simulink library "tqd"  (R2021b)
settings: Solver=VariableStepAuto  StartTime=0.0  StopTime=10.0  RelTol=1e-3
undefined symbols (not defined in the file or in its folder): ATQD_APSDecReq_X_kph, ATQD_APSDecReq_Y_mps2, ATQD_APSDecReqCMD_X_kph, ATQD_APSDecReqTs_X_pct, ATQD_APSDecTimeGain_X_Deg, ATQD_APSDecTimeGain_Y_s, ATQD_APSReqLowSpd_X_Deg, ATQD_AutoHoldReleaseBPS_X_Deg, ATQD_AWDLoadTrqnsGain_X_kg, ATQD_AWDLoadTrqnsGain_Y_pct, ATQD_BOSEnBPSPosn_X_kph, ATQD_BOSMap_X_rpm, ATQD_BOSMap_Y_pct, ATQD_CreepBaseTqD_X_kph, ATQD_CreepBaseTqD_Y_Deg, ATQD_CreepBaseTqR_X_kph, ATQD_CreepBaseTqR_Y_Deg, ATQD_CreepBPSDisPosn_X_Deg, ATQD_CreepBPSDisPosnR_X_Deg, ATQD_CreepBPSEnPosn_X_Deg, ATQD_CreepBPSEnPosnR_X_Deg, ATQD_CreepDeltaTq_X_kph, ATQD_CreepIterm_X_kph, ATQD_CreepIterm_Y_kph, ATQD_CreepItermMaxLimit_X_pct, ATQD_CreepPreloadTime_X_kph, ATQD_CreepPreloadTq_X_kph, ATQD_CreepPreloadTq_Y_s, ATQD_CreepProtTq_X_Deg, ATQD_CreepPterm_X_kph, ATQD_ECOTqMapD_X_rpm, ATQD_ECOTqMapD_Y_pct, ATQD_EOPDTqMapDCon_X_rpm, ATQD_EOPDTqMapDCon_Y_Deg, ATQD_EstInitVehWeight_X_c, ATQD_LHMRollGenMapD_X_rpm, ATQD_LHMRollGenMapD_Y_rpm, ATQD_LHMTqMapD_X_rpm, ATQD_LHMTqMapD_Y_pct, ATQD_NL1TqMapD_X_rpm, ATQD_NL1TqMapD_Y_pct, ATQD_NOPDTqMapDCon_X_rpm, ATQD_NOPDTqMapDCon_Y_Deg, ATQD_NRMRrEDUSpRat_X_rpm, ATQD_NRMRrEDUSpRat_Y_Nm, ATQD_OPDHoldDownRelDelay_X_Deg, ATQD_OPDHoldEnSpd_X_Deg, ATQD_OPDHoldRelDetTime_X_Deg, ATQD_OPDHoldReleaseTq_X_Deg, ATQD_OrigPedTqLowLim_X_Deg, ATQD_OrigPedTqLowLim_Y_pct, ATQD_PedalMapClimbUpLim_X_rpm, ATQD_PedalMapClimbUpLim_Y_Deg, ATQD_PreLoadTq_X_s, ATQD_RollGenMapEL1_X_rpm, ATQD_RollGenMapEL1_Y_rpm, ATQD_SL1TqMapD_X_rpm, ATQD_SL1TqMapD_Y_pct, ATQD_SlideRegenTqGain_X_Gps, ATQD_SlideRegenTqGain_Y_pct ... (+444)
libraries: hcu_lib x70, simulink x61, tqr x1
(part 10 of 14)

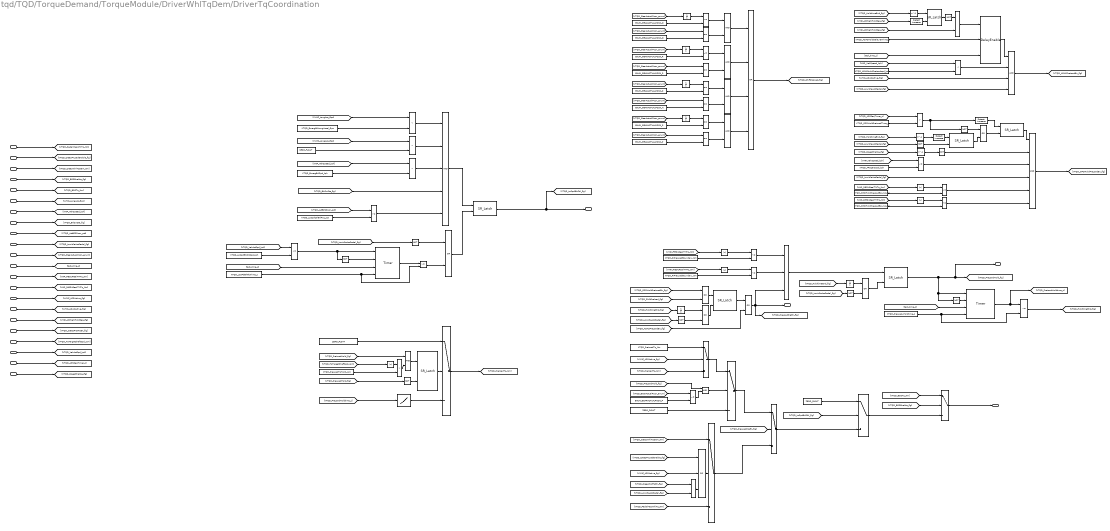
== system tqd/TQD/TorqueDemand/TorqueModule/DriverWhlTqDem/DriverTqCoordination ==
  VTQD_PedalMapWhlTq_Nm : Inport
  VTQD_CreepPrLoadEnable_flg : Inport  Port=2
  VTQD_CreepWhlTqDem_Nm : Inport  Port=3
  VTQD_BOSEnable_flg : Inport  Port=4
  VTQD_BOSTq_Nm : Inport  Port=5
  VVMC_LongAcc_Gps : Inport  Port=6
  VINP_VehSpeed_kph : Inport  Port=7
  VTQD_BrkSwSta_flg : Inport  Port=8
  VTQD_ActBPSPosn_pct : Inport  Port=9
  VTQD_LowIdleAccPedal_flg : Inport  Port=10
  VTQD_GearActualPosn_enum : Inport  Port=11
  task_time_s : Inport  Port=12
  VINP_FrEDURealTMTq_Nm : Inport  Port=13
  VINP_RrEDURealTMTq_Nm : Inport  Port=14
  VVMC_APSActive_flg : Inport  Port=15
  VVMC_ADASActive_flg : Inport  Port=16
  VINP_ACCVehHoldReq_flg : Inport  Port=17
  VTQD_CreepProtTqEn_flg : Inport  Port=18
  VTQD_TqTargetShaftSpd_rpm : Inport  Port=19
  VTQD_VehActSpd_kph : Inport  Port=20
  VTQD_APSReqTimer_s : Inport  Port=21
  VTQD_CreepEnable_flg : Inport  Port=22
  AND : Logic  Inputs=3  AllPortsSameDT=off  OutDataTypeStr=boolean
  AND{1..3,7..10} (7 alike) : Logic  AllPortsSameDT=off  OutDataTypeStr=boolean
  AND4 : Logic  Inputs=6  AllPortsSameDT=off  OutDataTypeStr=boolean
  AND5 : Logic  Inputs=4  AllPortsSameDT=off  OutDataTypeStr=boolean
  AND6 : Logic  Inputs=5  AllPortsSameDT=off  OutDataTypeStr=boolean
  Abs{,1..4} (5 alike) : Abs
  Constant : Constant  Value=KTQD_LoSpdCtrlBrkPos_pct
  Constant1 : Constant  Value=KTQD_RrPreLoadBoundary_Nm
  Constant{2,10,15,17} (4 alike) : Constant  Value=ZERO_FLOAT
  Constant11 : Constant  Value=KTQD_ADASHoldPreLoadspd_kph
  Constant12 : Constant  Value=KTQD_ADASHoldDelayEnTime_s
  Constant13 : Constant  Value=KTQD_EmergBrkSpd_kph
  Constant14 : Constant  Value=KTQD_EmergBrkLongAccel_Gps
  Constant16 : Constant  Value=KTQD_PreLoadTqHold_rpm
  Constant18 : Constant  Value=KTQD_OPDHoldPreLoadTime_s
  Constant19 : Constant  Value=KTQD_PreLoad_Holdtime_s
  Constant20 : Constant  Value=KTQD_APSZeroSpd_kph
  Constant21 : Constant  Value=ENUM_GEARACTUALPOSN_D
  Constant22 : Constant  Value=ENUM_GEARACTUALPOSN_D
  Constant{4,6,23..24} (4 alike) : Constant  Value=ENUM_GEARACTUALPOSN_R
  Constant25 : Constant  Value=KTQD_LoSPdBrkRlsTime_s
  Constant26 : Constant  Value=KTQD_LoSpdBrkRlsSpd_kph
  Constant27 : Constant  Value=KTQD_OPDHoldPreLoadBound_Nm
  Constant28 : Constant  Value=KTQD_OPDHoldPreLoadBound_Nm
  Constant3 : Constant  Value=KTQD_RrPreLoadBoundary_Nm
  Constant5 : Constant  Value=ENUM_GEARACTUALPOSN_N
  Constant7 : Constant  Value=ENUM_GEARACTUALPOSN_P
  Constant8 : Constant  Value=ENUM_GEARACTUALPOSN_P
  Constant9 : Constant  Value=KTQD_PreLoadTq_Nm
  Delay : Delay  DelayLength=1
  Delay1 : Delay  DelayLength=1
  Delay2 : Delay  DelayLength=1
  DelayEnable : hcu_lib/Basic_Blocks/DelayEnable
  Detect Increase : simulink/Logic and Bit Operations/Detect Increase  vinit=0.0  OutDataTypeStr=boolean
  Detect Increase1 : simulink/Logic and Bit Operations/Detect Increase  vinit=0.0  OutDataTypeStr=boolean
  Detect Increase2 : simulink/Logic and Bit Operations/Detect Increase  vinit=0.0  OutDataTypeStr=boolean
  Equal{1..4,6,8} (6 alike) : RelationalOperator  Operator===  OutDataTypeStr=boolean  RndMeth=Simplest
  Equal5 : RelationalOperator  Operator=~=  OutDataTypeStr=boolean  RndMeth=Simplest
  Equal7 : RelationalOperator  Operator=~=  OutDataTypeStr=boolean  RndMeth=Simplest
  Equal9 : RelationalOperator  Operator=~=  OutDataTypeStr=boolean  RndMeth=Simplest
  GreaterThan : RelationalOperator  OutDataTypeStr=boolean  RndMeth=Simplest
  Logical Operator : Logic  AllPortsSameDT=off  OutDataTypeStr=boolean
  MTQD_PreLoadTq_Y_Nm1 : Lookup_n-D  NumberOfTableDimensions=1  BreakpointsForDimension1=ATQD_PreLoadTq_X_s  Table=MTQD_PreLoadTq_Y_Nm  ExtrapMethod=Clip  InternalRulePriority=Speed  RndMeth=Simplest  InputSameDT=on
  NOT{,1..9} (10 alike) : Logic  Operator=NOT  AllPortsSameDT=off  OutDataTypeStr=boolean
  OR : Logic  Operator=OR  Inputs=3  AllPortsSameDT=off  OutDataTypeStr=boolean
  OR{1..2,4..7} (6 alike) : Logic  Operator=OR  AllPortsSameDT=off  OutDataTypeStr=boolean
  OR3 : Logic  Operator=OR  Inputs=4  AllPortsSameDT=off  OutDataTypeStr=boolean
  Relational Operator : RelationalOperator  OutDataTypeStr=boolean  RndMeth=Simplest
  Relational Operator{1..2,6,11..13} (6 alike) : RelationalOperator  Operator=<=  OutDataTypeStr=boolean  RndMeth=Simplest
  Relational Operator{3,8..10} (4 alike) : RelationalOperator  Operator=<  OutDataTypeStr=boolean  RndMeth=Simplest
  Relational Operator4 : RelationalOperator  Operator=>  OutDataTypeStr=boolean  RndMeth=Simplest
  Relational Operator5 : RelationalOperator  Operator=>  OutDataTypeStr=boolean  RndMeth=Simplest
  Relational Operator7 : RelationalOperator  OutDataTypeStr=boolean  RndMeth=Simplest
  SR_Latch{,1..6} (7 alike) : hcu_lib/Basic_Blocks/SR_Latch
  Switch{,1..4} (5 alike) : Switch  Criteria=u2 ~= 0
      Switch1 settings: AttributesFormatString=<%<Criteria>>
      Switch2 settings: AttributesFormatString=<%<Criteria>>
  Switch5 : Switch  Criteria=u2 > Threshold
  Switch6 : Switch  Criteria=u2 > Threshold
  Timer : hcu_lib/Basic_Blocks/Timer
  Timer1 : hcu_lib/Basic_Blocks/Timer
  Unit Delay{1..6} (6 alike) : UnitDelay  SampleTime=-1  HasFrameUpgradeWarning=on
  VTQD_DriverWhlTqDem_Nm : Outport
  VTQD_LoSpdBrkCtrl_flg : Outport  Port=2
  VTQD_PreLoadHold_flg : Outport  Port=3
  VTQD_PreLoadPreEn_flg : Outport  Port=4
  wires:
  VTQD_PedalMapWhlTq_Nm/1 -> [VTQD_PedalMapWhlTq_Nm]
  VTQD_CreepPrLoadEnable_flg/1 -> [VTQD_CreepPrLoadEnable_flg]
  VTQD_CreepWhlTqDem_Nm/1 -> [VTQD_CreepWhlTqDem_Nm]
  VTQD_BOSEnable_flg/1 -> [VTQD_BOSEnable_flg]
  VTQD_BOSTq_Nm/1 -> [VTQD_BOSTq_Nm]
  [VTQD_BOSEnable_flg] -> Switch1/2
  [VTQD_PedalMapWhlTq_Nm] -> Switch2/3
  [VTQD_CreepWhlTqDem_Nm] -> Switch2/1
  [VTQD_ActBPSPosn_pct] -> Relational Operator/1
  Constant/1 -> Relational Operator/2
  SR_Latch/1 -> [VTQD_LoSpdBrkCtrl_flg], VTQD_LoSpdBrkCtrl_flg/1  "VTQD_LoSpdBrkCtrl_flg"
  Constant10/1 -> Switch/1
  Switch1/1 -> VTQD_DriverWhlTqDem_Nm/1  "VTQD_DriverWhlTqDem_Nm"
  Switch/1 -> Switch1/3
  [VTQD_LowIdleAccPedal_flg] -> NOT/1
  [VTQD_VehActSpd_kph] -> Relational Operator6/1
  Constant26/1 -> Relational Operator6/2
  Relational Operator6/1 -> Timer/1, NOT1/1
  Timer/1 -> Relational Operator7/1
  NOT/1 -> OR2/1
  Relational Operator7/1 -> OR2/2
  OR2/1 -> SR_Latch/2  "VTQD_LoBrkCtrlReset_flg"
  NOT1/1 -> Timer/2
  Constant13/1 -> Relational Operator10/2
  [VINP_VehSpeed_kph] -> Relational Operator10/1
  Constant15/1 -> Relational Operator9/2
  Constant14/1 -> Relational Operator8/2
  [VVMC_LongAcc_Gps] -> Relational Operator8/1
  Relational Operator10/1 -> AND6/3
  Relational Operator9/1 -> AND6/2
  Relational Operator8/1 -> AND6/1
  [task_time_s] -> Timer/3
  VVMC_LongAcc_Gps/1 -> [VVMC_LongAcc_Gps]
  VINP_VehSpeed_kph/1 -> [VINP_VehSpeed_kph]
  VTQD_BrkSwSta_flg/1 -> [VTQD_BrkSwSta_flg]
  VTQD_ActBPSPosn_pct/1 -> [VTQD_ActBPSPosn_pct]
  VTQD_LowIdleAccPedal_flg/1 -> [VTQD_LowIdleAccPedal_flg]
  VTQD_GearActualPosn_enum/1 -> [VTQD_GearActualPosn_enum]
  task_time_s/1 -> [task_time_s]
  Constant25/1 -> Relational Operator7/2, Timer/4
  AND6/1 -> SR_Latch/1  "VTQD_TestLoSpdBrkCtrl_flg"
  [VTQD_BrkSwSta_flg] -> AND6/4
  Relational Operator/1 -> AND6/5
  Timer1/1 -> [VTQD_PreLoadHoldtime_s], GreaterThan/1  "VTQD_PreLoadHoldtime_s"
  GreaterThan/1 -> [VTQD_HoldtimeEnd_flg]  "VTQD_HoldtimeEnd_flg"
  [VTQD_PreLoadPreEn_flg] -> Switch4/2
  [VTQD_HoldtimeEnd_flg] -> Unit Delay4/1
  Constant19/1 -> GreaterThan/2, Timer1/4
  [task_time_s] -> Timer1/3
  Unit Delay2/1 -> Equal5/1
  [VTQD_GearActualPosn_enum] -> Unit Delay2/1
  Constant23/1 -> Equal7/2
  [VTQD_GearActualPosn_enum] -> Equal8/1
  Equal5/1 -> AND8/1
  AND9/1 -> OR3/2
  Constant21/1 -> Equal5/2
  Constant24/1 -> Equal8/2
  Unit Delay3/1 -> Equal7/1
  Constant22/1 -> Equal6/2
  AND8/1 -> OR3/1
  [VTQD_GearActualPosn_enum] -> Unit Delay3/1
  [VTQD_GearActualPosn_enum] -> Equal6/1
  Equal6/1 -> AND8/2
  Equal8/1 -> AND9/2
  OR3/1 -> [VTQD_ShiftPreload_flg]  "VTQD_ShiftPreload_flg"
  Equal7/1 -> AND9/1
  NOT2/1 -> Timer1/2
  Unit Delay4/1 -> OR4/1
  OR4/1 -> SR_Latch1/2
  Switch2/1 -> Switch4/3
  Switch4/1 -> Switch/3
  [VTQD_LowIdleAccPedal_flg] -> NOT3/1
  NOT3/1 -> OR4/2
  [VTQD_LoSpdBrkCtrl_flg] -> Switch/2
  VINP_FrEDURealTMTq_Nm/1 -> [VINP_FrEDURealTMTq_Nm]
  VINP_RrEDURealTMTq_Nm/1 -> [VINP_RrEDURealTMTq_Nm]
  [VTQD_GearActualPosn_enum] -> Equal2/1
  Constant5/1 -> Equal2/2
  Equal2/1 -> AND1/2
  Equal1/1 -> AND1/1
  Constant4/1 -> Equal1/2
  AND1/1 -> OR3/3
  [VTQD_GearActualPosn_enum] -> Unit Delay1/1
  Unit Delay1/1 -> Equal1/1
  Constant3/1 -> Relational Operator2/2
  Relational Operator2/1 -> AND/1
  Constant1/1 -> Relational Operator1/2
  Abs1/1 -> Relational Operator2/1
  Relational Operator1/1 -> AND/2
  Abs/1 -> Relational Operator1/1
  [VINP_RrEDURealTMTq_Nm] -> Abs/1
  [VINP_FrEDURealTMTq_Nm] -> Abs1/1
  OR5/1 -> AND/3, VTQD_PreLoadPreEn_flg/1, [VTQD_PreLoadPreEn_flg]  "VTQD_PreLoadPreEn_flg"
  Switch3/1 -> Switch4/1
  Constant2/1 -> Switch3/3
  Unit Delay5/1 -> Equal3/1
  [VTQD_GearActualPosn_enum] -> Unit Delay5/1
  Constant6/1 -> Equal3/2
  Equal3/1 -> AND2/1
  Equal4/1 -> AND2/2
  Constant7/1 -> Equal4/2
  [VTQD_GearActualPosn_enum] -> Equal4/1
  AND2/1 -> OR3/4
  AND/1 -> SR_Latch2/1
  NOT4/1 -> OR1/2
  [VTQD_LowIdleAccPedal_flg] -> NOT4/1
  Unit Delay6/1 -> OR1/1
  [VTQD_HoldtimeEnd_flg] -> Unit Delay6/1
  OR1/1 -> SR_Latch2/2
  [VTQD_GearActualPosn_enum] -> Equal9/1
  Constant8/1 -> Equal9/2
  Logical Operator/1 -> Switch3/2
  [VTQD_PreLoadHold_flg] -> Logical Operator/1
  Equal9/1 -> Logical Operator/2
  SR_Latch2/1 -> VTQD_PreLoadHold_flg/1, [VTQD_PreLoadHold_flg], NOT2/1, Timer1/1  "VTQD_PreLoadHold_flg"
  Constant12/1 -> DelayEnable/2
  Relational Operator3/1 -> AND5/2
  Constant11/1 -> Relational Operator3/2
  AND5/1 -> [VTQD_ADASPreLoadEn_flg]  "VTQD_ADASPreLoadEn_flg"
  AND7/1 -> DelayEnable/1  "VTQD_ADASPreLoadHold_flg"
  [VVMC_ADASActive_flg] -> AND5/3
  [VINP_ACCVehHoldReq_flg] -> Detect Increase/1
  Delay/1 -> SR_Latch3/1
  DelayEnable/1 -> AND5/1
  [VTQD_HoldtimeEnd_flg] -> Delay/1
  SR_Latch3/1 -> NOT5/1
  [VINP_ACCVehHoldReq_flg] -> AND7/2
  Detect Increase/1 -> SR_Latch3/2
  [task_time_s] -> DelayEnable/3  "task_time_s"
  [VINP_VehSpeed_kph] -> Relational Operator3/1
  NOT5/1 -> AND7/1
  Constant9/1 -> Switch5/1
  [VVMC_APSActive_flg] -> Switch5/2
  Switch5/1 -> Switch3/1
  [VVMC_APSActive_flg] -> OR/2
  OR/1 -> Switch2/2
  [VTQD_CreepPrLoadEnable_flg] -> OR/1
  [VTQD_ADASPreLoadEn_flg] -> OR5/2
  SR_Latch1/1 -> OR5/1
  VVMC_APSActive_flg/1 -> [VVMC_APSActive_flg]
  VVMC_ADASActive_flg/1 -> [VVMC_ADASActive_flg]
  VINP_ACCVehHoldReq_flg/1 -> [VINP_ACCVehHoldReq_flg]
  VTQD_CreepProtTqEn_flg/1 -> [VTQD_CreepProtTqEn_flg]
  [VTQD_CreepProtTqEn_flg] -> AND10/1
  [VTQD_LowIdleAccPedal_flg] -> AND10/2
  AND10/1 -> OR/3
  [VTQD_LowIdleAccPedal_flg] -> AND5/4
  [VTQD_PreLoadHold_flg] -> AND3/1
  Constant17/1 -> Switch6/1
  Abs2/1 -> Relational Operator4/1
  [VTQD_PreLoadHold_flg] -> NOT6/1
  [VTQD_TqTargetShaftSpd_rpm] -> Abs2/1
  Constant16/1 -> Relational Operator4/2
  NOT6/1 -> SR_Latch4/2
  Switch6/1 -> [VTQD_PreloadTq_Nm]  "VTQD_PreloadTq_Nm"
  SR_Latch4/1 -> Switch6/2
  MTQD_PreLoadTq_Y_Nm1/1 -> Switch6/3
  Relational Operator4/1 -> AND3/2
  AND3/1 -> SR_Latch4/1
  [VTQD_PreLoadHoldtime_s] -> MTQD_PreLoadTq_Y_Nm1/1
  [VTQD_PreloadTq_Nm] -> Switch5/3
  VTQD_TqTargetShaftSpd_rpm/1 -> [VTQD_TqTargetShaftSpd_rpm]
  [VTQD_BOSTq_Nm] -> Switch1/1
  VTQD_VehActSpd_kph/1 -> [VTQD_VehActSpd_kph]
  [VTQD_APSReqTimer_s] -> Relational Operator5/1
  Constant18/1 -> Relational Operator5/2
  Detect Increase1/1 -> SR_Latch5/1
  Relational Operator5/1 -> Detect Increase1/1, NOT8/1
  SR_Latch5/1 -> AND4/1
  AND4/1 -> [VTQD_OPDHoldPreLoadEn_flg]  "VTQD_OPDHoldPreLoadEn_flg"
  VTQD_APSReqTimer_s/1 -> [VTQD_APSReqTimer_s]
  VTQD_CreepEnable_flg/1 -> [VTQD_CreepEnable_flg]
  [VINP_VehSpeed_kph] -> Relational Operator11/1
  Constant20/1 -> Relational Operator11/2
  OR6/1 -> SR_Latch5/2
  NOT8/1 -> OR6/1
  NOT7/1 -> AND4/2
  Relational Operator11/1 -> AND4/3
  Delay2/1 -> NOT7/1
  [VTQD_CreepEnable_flg] -> Delay2/1
  Detect Increase2/1 -> SR_Latch6/1
  NOT9/1 -> SR_Latch6/2
  [VTQD_LowIdleAccPedal_flg] -> NOT9/1
  SR_Latch6/1 -> OR6/2
  Delay1/1 -> Detect Increase2/1
  [VTQD_HoldtimeEnd_flg] -> Delay1/1
  [VTQD_LowIdleAccPedal_flg] -> AND4/4
  Abs4/1 -> Relational Operator13/1
  Relational Operator12/1 -> AND4/6
  Constant28/1 -> Relational Operator13/2
  [VINP_FrEDURealTMTq_Nm] -> Abs4/1
  Relational Operator13/1 -> AND4/5
  Abs3/1 -> Relational Operator12/1
  [VINP_RrEDURealTMTq_Nm] -> Abs3/1
  Constant27/1 -> Relational Operator12/2
  [VVMC_LongAcc_Gps] -> Relational Operator9/1
  OR7/1 -> SR_Latch1/1
  [VTQD_ShiftPreload_flg] -> OR7/2
  [VTQD_OPDHoldPreLoadEn_flg] -> OR7/1

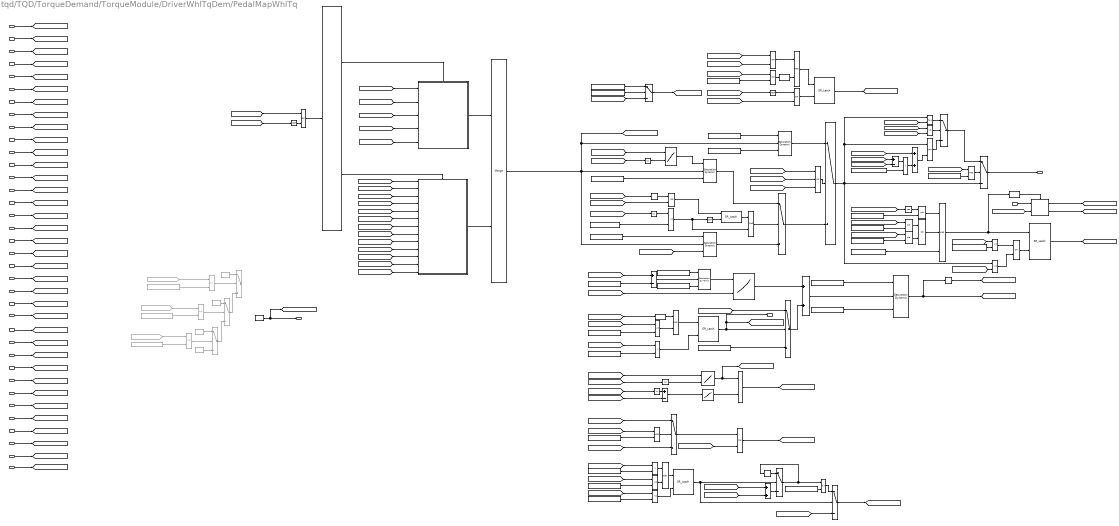
== system tqd/TQD/TorqueDemand/TorqueModule/DriverWhlTqDem/PedalMapWhlTq ==
  note: Driver Mode Valid Judge
  VTQD_GearActualPosn_enum : Inport
  VTQD_ActAPSPosn_pct : Inport  Port=2
  VTQD_TqTargetShaftSpd_rpm : Inport  Port=3
  VTQD_LimpHomeAct_flg : Inport  Port=4
  VTQD_EVDriveMode_enum : Inport  Port=5
  VTQD_RegenMode_enum : Inport  Port=6
  VTQD_RollRegenEnable_flg : Inport  Port=7
  VTQD_RollingShaftSpd_rpm : Inport  Port=8
  VTQD_RollRegenDisableReq_flg : Inport  Port=9
  VINP_HSAActive_flg : Inport  Port=10
  VVMC_ADASActive_flg : Inport  Port=11
  VVMC_ActMaxSlideRate_pct : Inport  Port=12
  VVMC_EstSlope_Deg : Inport  Port=13
  VVMC_LongAcc_Gps : Inport  Port=14
  VINP_SCPSystemMode_enum : Inport  Port=15
  VPMM_PwrSta_enum : Inport  Port=16
  VINP_SWCResUpSta_flg : Inport  Port=17
  task_time_s : Inport  Port=18
  VINP_VehSpeed_kph : Inport  Port=19
  VTQD_CreepPrLoadEnable_flg : Inport  Port=20
  VINP_BrkPedalPos_pct : Inport  Port=21
  VTQR_NoABSREDUWhlTqReq_Nm : Inport  Port=22
  VTQR_NoABSFEDUWhlTqReq_Nm : Inport  Port=23
  VINP_FrPTCSActive_flg : Inport  Port=24
  VINP_RrPTCSActive_flg : Inport  Port=25
  VINP_ADASACCSta_enum : Inport  Port=26
  VTQD_LowIdleAccPedal_flg : Inport  Port=27
  VTQD_BrkSwSta_flg : Inport  Port=28
  VTQD_OPDHoldEnRel_flg : Inport  Port=29
  VINP_SASAngle_Deg : Inport  Port=30
  VINP_YawRate_degps : Inport  Port=31
  VVMC_ActStESCYaw_degps : Inport  Port=32
  VTQD_APSReqTimer_s : Inport  Port=33
  VVMC_ACCOvrdMemTq_Nm : Inport  Port=34
  VVMC_LastADASWhlTqReq_Nm : Inport  Port=35
  VTQD_OPDHoldActRelTq_Nm : Inport  Port=36
  VTQD_VehActSpd_kph : Inport  Port=37
  AND{,1..4,6} (6 alike) : Logic  AllPortsSameDT=off  OutDataTypeStr=boolean
  AND5 : Logic  Inputs=3  AllPortsSameDT=off  OutDataTypeStr=boolean
  Abs{,1..3} (4 alike) : Abs
  Add : Sum  Inputs=+-
  Add1 : Sum
  Add13 : Sum  Inputs=+-
  Add2 : Sum
  Add3 : Sum
  Add4 : Sum  Inputs=+-
  Constant : Constant  Commented=on  Value=FALSE
  Constant1 : Constant  Commented=on  Value=ENUM_DRIVEMODE_NRM
  Constant10 : Constant  Value=KTQD_ClimbMin_rpm
  Constant11 : Constant  Value=KTQD_PedalMapRDCUpLim_Nm
  Constant12 : Constant  Value=KTQD_PedalMapRDCLowLim_Nm
  Constant13 : Constant  Value=KTQD_GRADE_Deg_ovrdval
  Constant14 : Constant  Value=KTQD_PedalMapRDCUpLim_Nm
  Constant15 : Constant  Value=KTQD_TargetSlideRate_pct
  Constant16 : Constant  Value=KTQD_SlideRateDevUpLim_pct
  Constant17 : Constant  Value=KTQD_SlideRateDevLowLim_pct
  Constant18 : Constant  Value=KTQD_PedalMapRDCLowLim_Nm
  Constant19 : Constant  Value=KTQD_SlideRegEnLimitTq_Nm
  Constant2 : Constant  Value=TRUE
  Constant20 : Constant  Value=KTQD_SlideRegEnLimitTq_Nm
  Constant21 : Constant  Value=KTQD_OrigPedTqLowLimSW_flg
  Constant22 : Constant  Value=KTQD_PedalMapRDCLowLim_Nm
  Constant23 : Constant  Value=KTQD_SlideRegenLowLim_Nm
  Constant24 : Constant  Value=KTQD_RgnEnLatchBrkPos_pct
  Constant25 : Constant  Value=ENUM_ADASACCSTA_SHUTOFF
  Constant26 : Constant  Value=KTQD_RgnEnLatchBrkPos_pct
  Constant27 : Constant  Value=KTQD_RgnEnLatchSlope_Deg
  Constant28 : Constant  Value=ZERO_FLOAT
  Constant29 : Constant  Value=ENUM_ADASACCSTA_STANDBY
  Constant3 : Constant  Commented=on  Value=TRUE
  Constant30 : Constant  Value=ENUM_ADASACCSTA_OFF
  Constant31 : Constant  Value=KTQD_ACCOvrdCancelResPedalTq_pct
  Constant32 : Constant  Value=KTQD_ACCOvrdCancelTqCtrl_flg
  Constant33 : Constant  Value=KVMC_ACCOvrdTestSW_flg
  Constant4 : Constant  Value=KTQD_GRADE_Deg_ovrdflg
  Constant5 : Constant  Value=KTQD_PedalMapClimbLowLim_Nm
  Constant6 : Constant  Commented=on  Value=ENUM_DRIVEMODE_ECO
  Constant69 : Constant  Value=KTQD_ACCOvrdCancelPedalTqRatio_Nm
  Constant7 : Constant  Commented=on  Value=ENUM_DRIVEMODE_SPORT
  Constant72 : Constant  Value=ENUM_ADASACCSTA_OVERRIDE
  Constant8 : Constant  Commented=on  Value=TRUE
  Constant9 : Constant  Commented=on  Value=TRUE
  Delay : Delay  DelayLength=1
  Delay1 : Delay  DelayLength=1
  Delay2 : Delay  DelayLength=1
  Detect Decrease : simulink/Logic and Bit Operations/Detect Decrease  vinit=0.0  OutDataTypeStr=boolean
  Detect Increase : simulink/Logic and Bit Operations/Detect Increase  vinit=0.0  OutDataTypeStr=boolean
  Detect Increase1 : simulink/Logic and Bit Operations/Detect Increase  vinit=0.0  OutDataTypeStr=boolean
  Divide7 : Product  Inputs=**
  Equal : RelationalOperator  Operator===  OutDataTypeStr=boolean  RndMeth=Simplest
  Equal3 : RelationalOperator  Commented=on  Operator===  OutDataTypeStr=boolean  RndMeth=Simplest
  Equal4 : RelationalOperator  Commented=on  Operator===  OutDataTypeStr=boolean  RndMeth=Simplest
  Equal5 : RelationalOperator  Commented=on  Operator===  OutDataTypeStr=boolean  RndMeth=Simplest
  From16 : From  Commented=on  GotoTag=VTQD_EVDriveMode_enum
  From17 : From  Commented=on  GotoTag=VTQD_EVDriveMode_enum
  From18 : From  Commented=on  GotoTag=VTQD_EVDriveMode_enum
  GearShiftCheck : If  IfExpression=u1~= 0
  LHM : Subsystem  TreatAsAtomicUnit=on
  Logical Operator : Logic  Operator=OR  AllPortsSameDT=off  OutDataTypeStr=boolean
  Logical Operator1 : Logic  Operator=NOT  AllPortsSameDT=off  OutDataTypeStr=boolean
  Logical Operator2 : Logic  Operator=OR  Inputs=3  AllPortsSameDT=off  OutDataTypeStr=boolean
  Logical Operator3 : Logic  Operator=OR  AllPortsSameDT=off  OutDataTypeStr=boolean
  MTQD_OrigPedTqLowLim_Z_Nm : Lookup_n-D  BreakpointsForDimension1=ATQD_OrigPedTqLowLim_Y_pct  BreakpointsForDimension2=ATQD_OrigPedTqLowLim_X_Deg  Table=MTQD_OrigPedTqLowLim_Z_Nm  ExtrapMethod=Clip  InternalRulePriority=Speed  RndMeth=Simplest  InputSameDT=on
      settings: InputPortMap=u0,u1
  MTQD_PedalMapClimbUpLim_Z_Nm : Lookup_n-D  BreakpointsForDimension1=ATQD_PedalMapClimbUpLim_Y_Deg  BreakpointsForDimension2=ATQD_PedalMapClimbUpLim_X_rpm  Table=MTQD_PedalMapClimbUpLim_Z_Nm  ExtrapMethod=Clip  InternalRulePriority=Speed  RndMeth=Simplest  InputSameDT=on
      settings: InputPortMap=u0,u1
  "MTQD_SlideRegenTqGain_Z_Nm " : Lookup_n-D  BreakpointsForDimension1=ATQD_SlideRegenTqGain_Y_pct  BreakpointsForDimension2=ATQD_SlideRegenTqGain_X_Gps  Table=MTQD_SlideRegenTqGain_Z_Nm  ExtrapMethod=Clip  InternalRulePriority=Speed  RndMeth=Simplest  InputSameDT=on
      settings: InputPortMap=u0,u1
  MTQD_YawTqLowLim_Y_Nm : Lookup_n-D  NumberOfTableDimensions=1  BreakpointsForDimension1=ATQD_YawTqLowLim_X_degps  Table=MTQD_YawTqLowLim_Y_Nm  ExtrapMethod=Clip  InternalRulePriority=Speed  RndMeth=Simplest  InputSameDT=on
  Max{,1..3} (4 alike) : MinMax  Function=max  Inputs=2
  Merge : Merge
  Min : MinMax  Inputs=2
  NOT : Logic  Operator=NOT  AllPortsSameDT=off  OutDataTypeStr=boolean
  NOT1 : Logic  Operator=NOT  AllPortsSameDT=off  OutDataTypeStr=boolean
  NoLHM : Subsystem  TreatAsAtomicUnit=on
  OR{,1..3} (4 alike) : Logic  Operator=OR  AllPortsSameDT=off  OutDataTypeStr=boolean
  Relational Operator{,1,3,6,9} (5 alike) : RelationalOperator  Operator=<=  OutDataTypeStr=boolean  RndMeth=Simplest
  Relational Operator10 : RelationalOperator  OutDataTypeStr=boolean  RndMeth=Simplest
  Relational Operator11 : RelationalOperator  OutDataTypeStr=boolean  RndMeth=Simplest
  Relational Operator2 : RelationalOperator  Operator=>  OutDataTypeStr=boolean  RndMeth=Simplest
  Relational Operator4 : RelationalOperator  Operator===  OutDataTypeStr=boolean  RndMeth=Simplest
  Relational Operator5 : RelationalOperator  Operator=>  OutDataTypeStr=boolean  RndMeth=Simplest
  Relational Operator7 : RelationalOperator  Operator===  OutDataTypeStr=boolean  RndMeth=Simplest
  Relational Operator8 : RelationalOperator  Operator===  OutDataTypeStr=boolean  RndMeth=Simplest
  SR_Latch{,1..4} (5 alike) : hcu_lib/Basic_Blocks/SR_Latch
  Saturation Dynamic{,1..4} (5 alike) : simulink/Discontinuities/Saturation Dynamic  OutMin=[]  OutMax=[]  OutDataTypeStr=Inherit: Same as second input  OutDataType=fixdt(1, 16)  OutScaling=2^-10  DoSatur=off
  Switch : Switch  Commented=on  Criteria=u2 ~= 0
      settings: AttributesFormatString=<%<Criteria>>
  Switch1 : Switch  Commented=on  Criteria=u2 ~= 0
      settings: AttributesFormatString=<%<Criteria>>
  Switch{6..11} (6 alike) : Switch  Criteria=u2 > Threshold
  Switch2 : Switch  Commented=on  Criteria=u2 ~= 0
      settings: AttributesFormatString=<%<Criteria>>
  Switch3 : Switch  Criteria=u2 ~= 0
  Switch4 : Switch  Criteria=u2 ~= 0
  Switch5 : Switch  Criteria=u2 ~= 0
  Triggered Subsystem : Subsystem  TreatAsAtomicUnit=on
  Unit Delay : UnitDelay  SampleTime=-1  HasFrameUpgradeWarning=on
  VTQD_PedalMapWhlTq_Nm : Outport
  VTQD_EVDriveModeValid_flg : Outport  Port=2
  VTQD_RegenTqLimitEn_flg : Outport  Port=3
  wires:
  [VTQD_GearActualPosn_enum] -> LHM/5(VTQD_GearActualPosn_enum)
  LHM/1(VTQD_PedalMapWhlTqLHM_Nm) -> Merge/1
  NoLHM/1(VTQD_PedalMapWhlTqNoLHM_Nm) -> Merge/2
  [VTQD_EVDriveMode_enum] -> NoLHM/7(VTQD_EVDriveMode_enum)
  [VTQD_GearActualPosn_enum] -> NoLHM/6(VTQD_GearActualPosn_enum)
  GearShiftCheck/2 -> NoLHM/Action
  GearShiftCheck/1 -> LHM/Action
  Logical Operator1/1 -> Logical Operator/2
  [VTQD_LimpHomeAct_flg] -> Logical Operator/1
  [VTQD_EVDriveModeValid_flg] -> Logical Operator1/1
  Logical Operator/1 -> GearShiftCheck/1
  Constant/1 -> Switch/3
  Constant3/1 -> Switch/1
  Constant2/1 -> [VTQD_EVDriveModeValid_flg], VTQD_EVDriveModeValid_flg/1  "VTQD_EVDriveModeValid_flg"
  Constant9/1 -> Switch2/1
  Switch1/1 -> Switch2/3
  Equal5/1 -> Switch2/2
  Constant7/1 -> Equal5/2
  From18/1 -> Equal5/1
  Constant8/1 -> Switch1/1
  Switch/1 -> Switch1/3
  Constant6/1 -> Equal4/2
  From17/1 -> Equal4/1
  Equal4/1 -> Switch1/2
  Equal3/1 -> Switch/2
  Constant1/1 -> Equal3/2
  From16/1 -> Equal3/1
  [VTQD_RollingShaftSpd_rpm] -> NoLHM/5(VTQD_RollingShaftSpd_rpm)
  [VTQD_RollRegenEnable_flg] -> NoLHM/4(VTQD_RollRegenEnable_flg)
  [VTQD_RollRegenEnable_flg] -> LHM/3(VTQD_RollRegenEnable_flg)
  [VTQD_RollingShaftSpd_rpm] -> LHM/4(VTQD_RollingShaftSpd_rpm)
  VTQD_RollingShaftSpd_rpm/1 -> [VTQD_RollingShaftSpd_rpm]
  VTQD_RollRegenEnable_flg/1 -> [VTQD_RollRegenEnable_flg]
  VTQD_RegenMode_enum/1 -> [VTQD_RegenMode_enum]
  VTQD_ActAPSPosn_pct/1 -> [VTQD_ActAPSPosn_pct]
  VTQD_EVDriveMode_enum/1 -> [VTQD_EVDriveMode_enum]
  VTQD_LimpHomeAct_flg/1 -> [VTQD_LimpHomeAct_flg]
  VTQD_GearActualPosn_enum/1 -> [VTQD_GearActualPosn_enum]
  VTQD_TqTargetShaftSpd_rpm/1 -> [VTQD_TqTargetShaftSpd_rpm]
  [VTQD_TqTargetShaftSpd_rpm] -> NoLHM/2(VTQD_TqTargetShaftSpd_rpm)
  [VTQD_RegenMode_enum] -> NoLHM/3(VTQD_RegenMode_enum)
  [VTQD_ActAPSPosn_pct] -> NoLHM/1(VTQD_ActAPSPosn_pct)
  [VTQD_ActAPSPosn_pct] -> LHM/1(VTQD_ActAPSPosn_pct)
  [VTQD_TqTargetShaftSpd_rpm] -> LHM/2(VTQD_TqTargetShaftSpd_rpm)
  VTQD_RollRegenDisableReq_flg/1 -> [VTQD_RollRegenDisableReq_flg]
  VINP_HSAActive_flg/1 -> [VINP_HSAActive_flg]
  Switch5/1 -> [VTQD_GRADE_Deg]  "VTQD_GRADE_Deg"
  Constant4/1 -> Switch5/2
  Constant13/1 -> Switch5/1
  Switch3/1 -> Switch4/3
  [VTQD_TqTargetShaftSpd_rpm] -> Abs/1
  Constant5/1 -> Saturation Dynamic/3
  SR_Latch/1 -> AND/1
  Relational Operator/1 -> AND/2, NOT/1
  Constant10/1 -> Relational Operator/2
  Constant12/1 -> Saturation Dynamic1/3
  Saturation Dynamic1/1 -> Switch4/1
  Saturation Dynamic/1 -> Switch3/1
  Abs/1 -> Relational Operator/1
  Abs1/1 -> MTQD_PedalMapClimbUpLim_Z_Nm/2
  [VTQD_TqTargetShaftSpd_rpm] -> Abs1/1
  AND/1 -> Switch3/2  "VTQD_ActHSAActive_flg"
  [VTQD_GRADE_Deg] -> MTQD_PedalMapClimbUpLim_Z_Nm/1
  NOT/1 -> SR_Latch/2
  MTQD_PedalMapClimbUpLim_Z_Nm/1 -> Saturation Dynamic/1  "VTQD_PedalMapClimbUpLim_Nm"
  Constant11/1 -> Saturation Dynamic1/1
  VVMC_ADASActive_flg/1 -> [VVMC_ADASActive_flg]
  Logical Operator2/1 -> Switch4/2
  Saturation Dynamic2/1 -> Switch3/3
  Constant14/1 -> Saturation Dynamic2/1
  VVMC_ActMaxSlideRate_pct/1 -> [VVMC_ActMaxSlideRate_pct]
  VVMC_LongAcc_Gps/1 -> [VVMC_LongAcc_Gps]
  VVMC_EstSlope_Deg/1 -> [VVMC_EstSlope_Deg]
  [VVMC_EstSlope_Deg] -> Switch5/3
  Constant21/1 -> AND2/2
  [VTQD_SlideRegenLimTq_Nm] -> Switch8/1
  [VTQD_RegenTqLimitEn_flg] -> AND2/1
  AND2/1 -> Switch8/2
  Add1/1 -> Saturation Dynamic4/2
  Detect Decrease/1 -> AND1/1
  Switch6/1 -> Add1/2
  [VVMC_LongAcc_Gps] -> "MTQD_SlideRegenTqGain_Z_Nm "/2
  Relational Operator2/1 -> SR_Latch1/2
  Constant18/1 -> Switch6/3
  Constant20/1 -> Relational Operator2/2
  [VTQD_RollRegenDisableReq_flg] -> Detect Decrease/1
  Add/1 -> Saturation Dynamic3/2
  Delay/1 -> [VTQD_LastSlideRegenLimTq_Nm]  "VTQD_LastSlideRegenLimTq_Nm"
  [VTQD_OrigPedalMapWhlTq_Nm] -> Relational Operator2/1
  Constant19/1 -> Relational Operator1/2
  SR_Latch1/1 -> VTQD_RegenTqLimitEn_flg/1, [VTQD_RegenTqLimitEn_flg], Switch6/2  "VTQD_RegenTqLimitEn_flg"
  "MTQD_SlideRegenTqGain_Z_Nm "/1 -> Add1/1  "VTQD_SlideRegenLimTqGain_Nm"
  Constant17/1 -> Saturation Dynamic3/3
  Constant23/1 -> Saturation Dynamic4/3
  [VVMC_ActMaxSlideRate_pct] -> Add/1
  [VTQD_OrigPedalMapWhlTq_Nm] -> Relational Operator1/1
  Relational Operator1/1 -> AND1/2
  Saturation Dynamic3/1 -> "MTQD_SlideRegenTqGain_Z_Nm "/1  "VTQD_SlideRateDev_pct"
  Saturation Dynamic4/1 -> Delay/1, [VTQD_SlideRegenLimTq_Nm]  "VTQD_SlideRegenLimTq_Nm"
  Constant15/1 -> Add/2
  Constant22/1 -> Saturation Dynamic4/1
  Constant16/1 -> Saturation Dynamic3/1
  AND1/1 -> SR_Latch1/1
  [VTQD_LastSlideRegenLimTq_Nm] -> Switch6/1
  VINP_RrPTCSActive_flg/1 -> [VINP_RrPTCSActive_flg]
  VINP_BrkPedalPos_pct/1 -> [VINP_BrkPedalPos_pct]
  VTQD_LowIdleAccPedal_flg/1 -> [VTQD_LowIdleAccPedal_flg]
  VINP_VehSpeed_kph/1 -> [VINP_VehSpeed_kph]
  VTQD_BrkSwSta_flg/1 -> [VTQD_BrkSwSta_flg]
  VINP_ADASACCSta_enum/1 -> [VINP_ADASACCSta_enum]
  VTQR_NoABSREDUWhlTqReq_Nm/1 -> [VTQR_NoABSREDUWhlTqReq_Nm]
  VTQR_NoABSFEDUWhlTqReq_Nm/1 -> [VTQR_NoABSFEDUWhlTqReq_Nm]
  VINP_FrPTCSActive_flg/1 -> [VINP_FrPTCSActive_flg]
  VPMM_PwrSta_enum/1 -> [VPMM_PwrSta_enum]
  VINP_SWCResUpSta_flg/1 -> [VINP_SWCResUpSta_flg]
  task_time_s/1 -> [task_time_s]
  VTQD_CreepPrLoadEnable_flg/1 -> [VTQD_CreepPrLoadEnable_flg]
  VINP_SCPSystemMode_enum/1 -> [VINP_SCPSystemMode_enum]
  Merge/1 -> Saturation Dynamic2/2, Saturation Dynamic/2, Saturation Dynamic1/2, [VTQD_OrigPedalMapWhlTq_Nm]  "VTQD_OrigPedalMapWhlTq_Nm"
  Equal/1 -> Detect Increase/1
  [VINP_FrPTCSActive_flg] -> Logical Operator3/2
  Logical Operator3/1 -> AND3/1
  AND3/1 -> SR_Latch3/1
  [VTQD_BrkSwSta_flg] -> OR/2
  Detect Increase/1 -> AND3/2
  NOT1/1 -> OR/1
  [VTQD_LowIdleAccPedal_flg] -> NOT1/1
  Constant25/1 -> Equal/2
  SR_Latch3/1 -> [VTQD_ADASShutOff_flg]  "VTQD_ADASShutOff_flg"
  OR/1 -> SR_Latch3/2
  [VINP_RrPTCSActive_flg] -> Logical Operator3/1
  [VVMC_ADASActive_flg] -> Logical Operator2/3
  [VTQD_RollRegenDisableReq_flg] -> Logical Operator2/2
  [VTQD_ADASShutOff_flg] -> Logical Operator2/1
  Max/1 -> [VTQD_OrigPedTqLowLim_Nm]  "VTQD_OrigPedTqLowLim_Nm"
  [VTQD_BrkRgnLatchTqLim_Nm] -> Max/2
  Switch8/1 -> Max/1
  [VTQD_OrigPedTqLowLim_Nm] -> Saturation Dynamic2/3
  [VTQD_SlideTqLowLim_Nm] -> Switch9/3
  Relational Operator3/1 -> SR_Latch2/2
  SR_Latch2/1 -> Switch9/2, Switch10/2
  [VTQR_NoABSFEDUWhlTqReq_Nm] -> Add2/2
  Constant27/1 -> Relational Operator6/2
  Constant24/1 -> Relational Operator3/2
  Switch9/1 -> [VTQD_BrkRgnLatchTqLim_Nm]  "VTQD_BrkRgnLatchTqLim_Nm"
  Constant26/1 -> Relational Operator5/2
  Min/1 -> Switch9/1
  [VINP_BrkPedalPos_pct] -> Relational Operator3/1
  Relational Operator6/1 -> AND4/2
  [VVMC_EstSlope_Deg] -> Relational Operator6/1
  [VTQR_NoABSREDUWhlTqReq_Nm] -> Add2/1
  AND4/1 -> SR_Latch2/1
  Switch10/1 -> Min/1, Delay2/1
  Relational Operator5/1 -> AND4/1
  Constant28/1 -> Min/2
  Delay2/1 -> Switch10/1
  [VINP_BrkPedalPos_pct] -> Relational Operator5/1
  Add2/1 -> Switch10/3
  [VINP_ADASACCSta_enum] -> Equal/1
  Switch7/1 -> VTQD_PedalMapWhlTq_Nm/1  "VTQD_PedalMapWhlTqTest_Nm"
  [VINP_HSAActive_flg] -> OR1/2
  OR1/1 -> SR_Latch/1
  VTQD_OPDHoldEnRel_flg/1 -> [VTQD_OPDHoldEnRel_flg]
  Delay1/1 -> OR1/1
  [VVMC_ActMaxSlideRate_pct] -> MTQD_OrigPedTqLowLim_Z_Nm/1
  [VINP_YawRate_degps] -> Abs2/1
  [VVMC_ActStESCYaw_degps] -> Add4/2
  Abs2/1 -> Add4/1
  Add4/1 -> MTQD_YawTqLowLim_Y_Nm/1  "VTQD_TqLowLimYawDev_degps"
  MTQD_OrigPedTqLowLim_Z_Nm/1 -> [VTQD_SlideTqLowLim_Nm], Max1/1  "VTQD_SlideTqLowLim_Nm"
  MTQD_YawTqLowLim_Y_Nm/1 -> Max1/2  "VTQD_YawTqLowLim_Nm"
  Max1/1 -> [VTQD_PreDecTqLowLim_Nm]  "VTQD_PreDecTqLowLim_Nm"
  [VTQD_PreDecTqLowLim_Nm] -> Switch8/3
  VINP_SASAngle_Deg/1 -> [VINP_SASAngle_Deg]
  VVMC_ActStESCYaw_degps/1 -> [VVMC_ActStESCYaw_degps]
  VINP_YawRate_degps/1 -> [VINP_YawRate_degps]
  Abs3/1 -> MTQD_OrigPedTqLowLim_Z_Nm/2
  [VINP_SASAngle_Deg] -> Abs3/1
  [VTQD_OPDHoldEnRel_flg] -> Delay1/1
  [VVMC_EstSlope_Deg] -> NoLHM/8(VVMC_EstSlope_Deg)
  [VTQD_APSReqTimer_s] -> NoLHM/9(VTQD_APSReqTimer_s)
  VTQD_APSReqTimer_s/1 -> [VTQD_APSReqTimer_s]
  [VTQD_LowIdleAccPedal_flg] -> NoLHM/10(VTQD_LowIdleAccPedal_flg)
  [VINP_ADASACCSta_enum] -> Unit Delay/1
  Constant72/1 -> Relational Operator4/2
  Unit Delay/1 -> Relational Operator4/1
  [VINP_ADASACCSta_enum] -> Relational Operator7/1
  Constant29/1 -> Relational Operator7/2
  Relational Operator7/1 -> OR2/1
  Relational Operator4/1 -> AND5/1
  AND5/1 -> Detect Increase1/1, SR_Latch4/1
  Constant30/1 -> Relational Operator8/2
  [VINP_ADASACCSta_enum] -> Relational Operator8/1
  Relational Operator8/1 -> OR2/2
  OR2/1 -> AND5/2
  SR_Latch4/1 -> [VTQD_ACCCancelDet_flg]  "VTQD_ACCCancelDet_flg"
  [VTQD_ACCCancelDet_flg] -> AND6/1
  Switch11/1 -> Switch7/1
  Switch4/1 -> Switch7/3, Max2/1, Max3/1, Relational Operator11/1  "VTQD_PedalMapWhlTq_Nm"
  VVMC_ACCOvrdMemTq_Nm/1 -> [VVMC_ACCOvrdMemTq_Nm]
  [VTQD_ActAPSPosn_pct] -> Relational Operator9/1
  Relational Operator9/1 -> OR3/1
  Constant31/1 -> Relational Operator9/2
  Constant32/1 -> AND5/3
  Detect Increase1/1 -> Triggered Subsystem/Trigger
  VVMC_LastADASWhlTqReq_Nm/1 -> Triggered Subsystem/1(in1)
  Triggered Subsystem/1(Out1) -> [VTQD_ACCCancelMemTq_Nm]  "VTQD_ACCCancelMemTq_Nm"
  [VTQD_ActAPSPosn_pct] -> Triggered Subsystem/2(In2)
  Triggered Subsystem/2(Out2) -> [VTQD_ACCCancelMemPosn_pct]  "VTQD_ACCCancelMemPosn_pct"
  [VTQD_ActAPSPosn_pct] -> Relational Operator10/1
  [VTQD_ACCCancelMemPosn_pct] -> Relational Operator10/2
  [VTQD_ACCCancelMemTq_Nm] -> Max2/2
  Relational Operator10/1 -> Switch11/2
  Max2/1 -> Switch11/1
  [VTQD_ActAPSPosn_pct] -> Add13/1
  [VTQD_ACCCancelMemPosn_pct] -> Add13/2
  Constant69/1 -> Divide7/2
  Add13/1 -> Divide7/1
  Divide7/1 -> Add3/2
  [VTQD_ACCCancelMemTq_Nm] -> Add3/1
  Max3/1 -> Switch11/3
  Add3/1 -> Max3/2
  [VTQD_ACCCancelMemTq_Nm] -> Relational Operator11/2
  Relational Operator11/1 -> OR3/2
  OR3/1 -> SR_Latch4/2
  AND6/1 -> Switch7/2
  Constant33/1 -> AND6/2
  [VTQD_OPDHoldEnRel_flg] -> NoLHM/11(VTQD_OPDHoldEnRel_flg)
  [VTQD_OPDHoldActRelTq_Nm] -> NoLHM/12(VTQD_OPDHoldActRelTq_Nm)
  [VTQD_VehActSpd_kph] -> NoLHM/13(VTQD_VehActSpd_kph)
  VTQD_OPDHoldActRelTq_Nm/1 -> [VTQD_OPDHoldActRelTq_Nm]
  VTQD_VehActSpd_kph/1 -> [VTQD_VehActSpd_kph]

== system tqd/TQD/TorqueDemand/TorqueModule/DriverWhlTqDem/RollingRegenJudge ==
  VDHP_LowIdleAccPedal_flg : Inport
  VINP_VehSpd_kph : Inport  Port=2
  VTQD_TqTargetShaftSpd_rpm : Inport  Port=3
  VTQD_RollRegenDisableReq_flg : Inport  Port=4
  VTQD_TqSourceFr_enum : Inport  Port=5
  VTQD_TqSourceRr_enum : Inport  Port=6
  VTQD_CreepEnable_flg : Inport  Port=7
  Constant : Constant  Value=ENUM_TQSOURCE_CC
  Constant1 : Constant  Value=ENUM_TQSOURCE_ADAS
  Constant2 : Constant  Value=ENUM_TQSOURCE_APS
  Constant3 : Constant  Value=ENUM_TQSOURCE_CC
  Constant4 : Constant  Value=ENUM_TQSOURCE_ADAS
  Constant5 : Constant  Value=ENUM_TQSOURCE_APS
  Detect Increase : simulink/Logic and Bit Operations/Detect Increase  vinit=0.0  OutDataTypeStr=boolean
  Equal{,1..5} (6 alike) : RelationalOperator  Operator===  OutDataTypeStr=boolean  RndMeth=Simplest
  Logical Operator : Logic  Inputs=5  AllPortsSameDT=off  OutDataTypeStr=boolean
  Logical Operator1 : Logic  Operator=NOT  AllPortsSameDT=off  OutDataTypeStr=boolean
  Logical Operator10 : Logic  Operator=OR  AllPortsSameDT=off  OutDataTypeStr=boolean
  Logical Operator11 : Logic  Operator=NOT  AllPortsSameDT=off  OutDataTypeStr=boolean
  Logical Operator12 : Logic  Operator=NOT  AllPortsSameDT=off  OutDataTypeStr=boolean
  Logical Operator5 : Logic  Operator=OR  Inputs=3  AllPortsSameDT=off  OutDataTypeStr=boolean
  Logical Operator9 : Logic  Operator=OR  Inputs=3  AllPortsSameDT=off  OutDataTypeStr=boolean
  Relay : Relay  OnSwitchValue=KTQD_RegenOnSpd_kph  OffSwitchValue=KTQD_RegenOffSpd_kph
      settings: AttributesFormatString=|
      | ON: %<OnSwitchValue>
      | OFF: %<OffSwitchValue>
  Switch2 : Switch  Criteria=u2 ~= 0
      settings: AttributesFormatString=<%<Criteria>>
  Unit Delay : UnitDelay  SampleTime=-1  HasFrameUpgradeWarning=on
  Unit Delay1 : UnitDelay  SampleTime=-1  HasFrameUpgradeWarning=on
  VTQD_RollRegenEnable_flg : Outport
  VTQD_RollingShaftSpd_rpm : Outport  Port=2
  wires:
  Equal5/1 -> Logical Operator9/3
  Equal3/1 -> Logical Operator9/1
  Equal4/1 -> Logical Operator9/2
  Constant4/1 -> Equal4/2
  [VTQD_TqSourceRr_enum] -> Equal4/1
  Constant5/1 -> Equal5/2
  [VTQD_TqSourceRr_enum] -> Equal5/1
  Constant3/1 -> Equal3/2
  [VTQD_TqSourceRr_enum] -> Equal3/1
  Constant2/1 -> Equal2/2
  [VTQD_TqSourceFr_enum] -> Equal2/1
  Constant1/1 -> Equal1/2
  [VTQD_TqSourceFr_enum] -> Equal1/1
  Constant/1 -> Equal/2
  Logical Operator11/1 -> Logical Operator/5
  Logical Operator10/1 -> Logical Operator11/1
  Logical Operator9/1 -> Logical Operator10/2
  Logical Operator5/1 -> Logical Operator10/1
  [VTQD_CreepEnable_flg] -> Unit Delay1/1
  Equal2/1 -> Logical Operator5/3
  Equal1/1 -> Logical Operator5/2
  Equal/1 -> Logical Operator5/1
  VTQD_CreepEnable_flg/1 -> [VTQD_CreepEnable_flg]
  VTQD_TqSourceFr_enum/1 -> [VTQD_TqSourceFr_enum]
  VTQD_TqSourceRr_enum/1 -> [VTQD_TqSourceRr_enum]
  [VTQD_RollRegenDisableReq_flg] -> Logical Operator1/1
  VTQD_RollRegenDisableReq_flg/1 -> [VTQD_RollRegenDisableReq_flg]
  Unit Delay/1 -> Switch2/3
  Switch2/1 -> VTQD_RollingShaftSpd_rpm/1, Unit Delay/1  "VTQD_RollingShaftSpd_rpm"
  [VTQD_TqTargetShaftSpd_rpm] -> Switch2/1
  Detect Increase/1 -> Switch2/2
  [VTQD_RollRegenEnable_flg] -> Detect Increase/1
  VTQD_TqTargetShaftSpd_rpm/1 -> [VTQD_TqTargetShaftSpd_rpm]
  [VINP_VehSpd_kph] -> Relay/1
  VINP_VehSpd_kph/1 -> [VINP_VehSpd_kph]
  VDHP_LowIdleAccPedal_flg/1 -> [VTQD_LowIdleAccPedal_flg]
  Logical Operator/1 -> VTQD_RollRegenEnable_flg/1, [VTQD_RollRegenEnable_flg]  "VTQD_RollRegenEnable_flg"
  Unit Delay1/1 -> Logical Operator12/1
  Relay/1 -> Logical Operator/2
  Logical Operator12/1 -> Logical Operator/4
  Logical Operator1/1 -> Logical Operator/3
  [VTQD_LowIdleAccPedal_flg] -> Logical Operator/1
  [VTQD_TqSourceFr_enum] -> Equal/1

== system tqd/TQD/TorqueDemand/TorqueModule/OPD Hold/Deceleration Calculation ==
  VTQD_VehActSpd_kph : Inport
  VVMC_LongAcc_Gps : Inport  Port=2
  VTQD_APSReqTimer_s : Inport  Port=3
  VVMC_EstSlope_Deg : Inport  Port=4
  VTQD_APSDecReqA_flg : Inport  Port=5
  VTQD_AutiHoldRelease_flg : Inport  Port=6
  task_time_s : Inport  Port=7
  VTQD_ActAPSPosn_pct : Inport  Port=8
  AND1 : Logic  Inputs=3  AllPortsSameDT=off  OutDataTypeStr=boolean
  AND4 : Logic  Inputs=3  AllPortsSameDT=off  OutDataTypeStr=boolean
  Add : Sum  Inputs=+-
  Constant1 : Constant  Value=KTQD_APSDecReqMaxTime_s
  Constant13 : Constant  Value=ZERO_FLOAT
  Constant19 : Constant  Value=KTQD_OPDHoldBrkSW_flg
  Constant2 : Constant  Value=KTQD_OPDHoldBrkSW_flg
  Constant21 : Constant  Value=KTQD_OPDHoldDevUpLim_mps2
  Constant22 : Constant  Value=KTQD_OPDHoldDevLowLim_mps2
  Constant43 : Constant  Value=KTQD_APSDecReqMaxSW_flg
  Constant8 : Constant  Value=KVMC_GravityValue_mps2
  Delay : Delay  DelayLength=1
  FirstOrderFilter1 : tqr/TQR/Determine Torque Request/TorqueArbitrament/TorqueSmooth/FirstOrderFilter
  MTQD_APSDecReg_Z_mps2 : Lookup_n-D  BreakpointsForDimension1=ATQD_APSDecReq_Y_mps2  BreakpointsForDimension2=ATQD_APSDecReq_X_kph  Table=MTQD_APSDecReq_Z_mps2  InternalRulePriority=Speed  RndMeth=Simplest  InputSameDT=on
      settings: InputPortMap=u0,u1
  MTQD_APSDecReqCMD_Y_mps2 : Lookup_n-D  NumberOfTableDimensions=1  BreakpointsForDimension1=ATQD_APSDecReqCMD_X_kph  Table=MTQD_APSDecReqCMD_Y_mps2  InternalRulePriority=Speed  RndMeth=Simplest  InputSameDT=on
  MTQD_APSDecReqTs_Y_c : Lookup_n-D  NumberOfTableDimensions=1  BreakpointsForDimension1=ATQD_APSDecReqTs_X_pct  Table=MTQD_APSDecReqTs_Y_c  InternalRulePriority=Speed  RndMeth=Simplest  InputSameDT=on
  MTQD_APSDecTimeGain_Z_c : Lookup_n-D  BreakpointsForDimension1=ATQD_APSDecTimeGain_Y_s  BreakpointsForDimension2=ATQD_APSDecTimeGain_X_Deg  Table=MTQD_APSDecTimeGain_Z_c  InternalRulePriority=Speed  RndMeth=Simplest  InputSameDT=on
      settings: InputPortMap=u0,u1
  Max : MinMax  Function=max  Inputs=2
  NOT{1..3,5} (4 alike) : Logic  Operator=NOT  AllPortsSameDT=off  OutDataTypeStr=boolean
  OR : Logic  Operator=OR  AllPortsSameDT=off  OutDataTypeStr=boolean
  Product : Product
  Product1 : Product
  Product2 : Product
  Relational Operator : RelationalOperator  OutDataTypeStr=boolean  RndMeth=Simplest
  SR_Latch : hcu_lib/Basic_Blocks/SR_Latch
  Saturation Dynamic : simulink/Discontinuities/Saturation Dynamic  OutMin=[]  OutMax=[]  OutDataTypeStr=Inherit: Same as second input  OutDataType=fixdt(1, 16)  OutScaling=2^-10  DoSatur=off
  Switch1 : Switch  Criteria=u2 > Threshold
  Switch3 : Switch  Criteria=u2 > Threshold
  Switch9 : Switch  Criteria=u2 > Threshold
  VTQD_APSDecReq_mps2 : Outport
  wires:
  Saturation Dynamic/1 -> MTQD_APSDecReg_Z_mps2/1  "VTQD_ActOPDHoldAccDev_mps2"
  [VVMC_EstSlope_Deg] -> MTQD_APSDecTimeGain_Z_c/2
  [VTQD_APSDecTimeGain_c] -> Product2/2
  Constant21/1 -> Saturation Dynamic/1
  Product/1 -> Max/1
  Max/1 -> Switch9/1
  MTQD_APSDecReg_Z_mps2/1 -> [VTQD_MapAPSDecReg_mps2]  "VTQD_MapAPSDecReq_mps2"
  Constant13/1 -> Switch3/3
  MTQD_APSDecReqCMD_Y_mps2/1 -> [VTQD_APSDecReqCMD_mps2]  "VTQD_APSDecReqCMD_mps2"
  [VVMC_LongAcc_Gps] -> Product1/1
  [VTQD_MapAPSDecReg_mps2] -> Product2/1
  Delay/1 -> Max/2
  Constant19/1 -> NOT5/1
  Add/1 -> Saturation Dynamic/2
  [VTQD_VehActSpd_kph] -> MTQD_APSDecReg_Z_mps2/2
  [VTQD_APSReqTimer_s] -> MTQD_APSDecTimeGain_Z_c/1
  [VTQD_MapAPSDecReg_mps2] -> Product/1
  Product2/1 -> Switch9/3
  [VTQD_APSDecReq_mps2] -> Delay/1
  Product1/1 -> Add/2
  [VTQD_VehActSpd_kph] -> MTQD_APSDecReqCMD_Y_mps2/1
  MTQD_APSDecTimeGain_Z_c/1 -> [VTQD_APSDecTimeGain_c]  "VTQD_APSDecTimeGain_c"
  [VTQD_APSDecReqA_flg] -> AND4/1
  NOT5/1 -> AND4/2
  [VTQD_APSDecTimeGain_c] -> Product/2
  [VTQD_APSDecReqCMD_mps2] -> Add/1
  Constant22/1 -> Saturation Dynamic/3
  Constant8/1 -> Product1/2
  VTQD_VehActSpd_kph/1 -> [VTQD_VehActSpd_kph]
  VVMC_LongAcc_Gps/1 -> [VVMC_LongAcc_Gps]
  VTQD_APSReqTimer_s/1 -> [VTQD_APSReqTimer_s]
  VVMC_EstSlope_Deg/1 -> [VVMC_EstSlope_Deg]
  VTQD_APSDecReqA_flg/1 -> [VTQD_APSDecReqA_flg]
  [VTQD_APSDecReq_mps2] -> VTQD_APSDecReq_mps2/1
  Constant43/1 -> OR/1
  Relational Operator/1 -> SR_Latch/1
  Constant1/1 -> Relational Operator/2
  [VTQD_APSReqTimer_s] -> Relational Operator/1
  Switch9/1 -> Switch3/1
  [VTQD_AutiHoldRelease_flg] -> SR_Latch/2
  VTQD_AutiHoldRelease_flg/1 -> [VTQD_AutiHoldRelease_flg]
  OR/1 -> Switch9/2  "VTQD_APSDecReqMax_flg"
  SR_Latch/1 -> OR/2
  AND4/1 -> Switch3/2
  NOT2/1 -> AND4/3
  [VTQD_AutiHoldRelease_flg] -> NOT2/1
  NOT1/1 -> AND1/3
  NOT3/1 -> AND1/2
  AND1/1 -> Switch1/2
  Switch3/1 -> Switch1/1, FirstOrderFilter1/1
  Switch1/1 -> [VTQD_APSDecReq_mps2]  "VTQD_APSDecReq_mps2"
  [VTQD_APSDecReqA_flg] -> AND1/1
  Constant2/1 -> NOT3/1
  [VTQD_AutiHoldRelease_flg] -> NOT1/1
  FirstOrderFilter1/1 -> Switch1/3
  [task_time_s] -> FirstOrderFilter1/2
  task_time_s/1 -> [task_time_s]
  VTQD_ActAPSPosn_pct/1 -> [VTQD_ActAPSPosn_pct]
  MTQD_APSDecReqTs_Y_c/1 -> [VTQD_APSDecReqTs_c]  "VTQD_APSDecReqTs_c"
  [VTQD_ActAPSPosn_pct] -> MTQD_APSDecReqTs_Y_c/1
  [VTQD_APSDecReqTs_c] -> FirstOrderFilter1/3

== system tqd/TQD/TorqueDemand/TorqueModule/OPD Hold/OPDHold Request  ==
  VTQD_VehActSpd_kph : Inport
  VTQD_APSStaSys_enum : Inport  Port=2
  VTQD_AutiHoldRelease_flg : Inport  Port=3
  task_time_s : Inport  Port=4
  VVMC_EstSlope_Deg : Inport  Port=5
  AND : Logic  AllPortsSameDT=off  OutDataTypeStr=boolean
  AND1 : Logic  Inputs=3  AllPortsSameDT=off  OutDataTypeStr=boolean
  AND2 : Logic  Operator=OR  AllPortsSameDT=off  OutDataTypeStr=boolean
  Constant1 : Constant  Value=KTQD_APSReqUpSpd_kph
  Constant10 : Constant  Value=KTQD_APSReqDownSpd_kph
  Constant11 : Constant  Value=ZERO_FLOAT  OutDataTypeStr=uint8
  Constant2 : Constant  Value=2  OutDataTypeStr=uint8
  Constant3 : Constant  Value=2  OutDataTypeStr=uint8
  Constant4 : Constant  OutDataTypeStr=uint8
  Constant5 : Constant  Value=2  OutDataTypeStr=uint8
  Constant6 : Constant  Value=0  OutDataTypeStr=uint8
  Constant7 : Constant  OutDataTypeStr=uint8
  Constant8 : Constant  OutDataTypeStr=uint8
  Constant9 : Constant  Value=KTQD_APSReqDelayTime_s
  Equal1 : RelationalOperator  Operator=<  OutDataTypeStr=boolean  RndMeth=Simplest
  Equal2 : RelationalOperator  Operator=~=  OutDataTypeStr=boolean  RndMeth=Simplest
  Equal3 : RelationalOperator  Operator===  OutDataTypeStr=boolean  RndMeth=Simplest
  Equal4 : RelationalOperator  Operator===  OutDataTypeStr=boolean  RndMeth=Simplest
  Equal5 : RelationalOperator  Operator===  OutDataTypeStr=boolean  RndMeth=Simplest
  Equal6 : RelationalOperator  Operator=>  OutDataTypeStr=boolean  RndMeth=Simplest
  MTQD_APSReqLowSpd_Y_kph : Lookup_n-D  NumberOfTableDimensions=1  BreakpointsForDimension1=ATQD_APSReqLowSpd_X_Deg  Table=MTQD_APSReqLowSpd_Y_kph  InternalRulePriority=Speed  RndMeth=Simplest  InputSameDT=on
  NOT1 : Logic  Operator=NOT  AllPortsSameDT=off  OutDataTypeStr=boolean
  NOT2 : Logic  Operator=NOT  AllPortsSameDT=off  OutDataTypeStr=boolean
  Relational Operator1 : RelationalOperator  Operator=<  OutDataTypeStr=boolean  RndMeth=Simplest
  Relational Operator2 : RelationalOperator  OutDataTypeStr=boolean  RndMeth=Simplest
  Relay : Relay  OnSwitchValue=KTQD_OPDHoldGradeUp_Deg  OffSwitchValue=KTQD_OPDHoldGradeDown_Deg  OutDataTypeStr=boolean
  SR_Latch : hcu_lib/Basic_Blocks/SR_Latch
  Switch : Switch  Criteria=u2 > Threshold
  Switch1 : Switch  Criteria=u2 > Threshold
  Switch2 : Switch  Criteria=u2 > Threshold
  Timer : hcu_lib/Basic_Blocks/Timer
  VTQD_APSReqTimer_s : Outport
  VTQD_APSReq_enum : Outport  Port=2
  VTQD_APSDecReqA_flg : Outport  Port=3
  VTQD_OPDHoldLamp_flg : Outport  Port=4
  wires:
  [task_time_s] -> Timer/3
  Constant4/1 -> Switch1/1
  NOT2/1 -> Timer/2
  Switch2/1 -> [VTQD_APSReq_enum]  "VTQD_APSReq_enum"
  AND/1 -> Switch1/2  "VTQD_APSStasysUp_flg"
  Constant9/1 -> Relational Operator2/2, Timer/4
  Equal3/1 -> AND/2
  Constant6/1 -> Switch1/3
  Timer/1 -> [VTQD_APSReqTimer_s], Relational Operator2/1  "VTQD_APSReqTimer_s"
  Relational Operator2/1 -> Switch2/2
  Constant8/1 -> Switch2/1
  Equal4/1 -> AND1/2
  [VTQD_APSStaSys_enum] -> Equal3/1
  [VTQD_VehActSpd_kph] -> Equal1/1
  Equal5/1 -> [VTQD_APSDecReqA_flg]  "VTQD_APSDecReqA_flg"
  [VTQD_APSReqUpSpd_kph] -> Equal1/2
  NOT1/1 -> AND1/3
  Constant7/1 -> Equal5/2
  [VTQD_APSReq_enum] -> Equal5/1
  Constant2/1 -> Equal3/2
  Switch1/1 -> Switch2/3
  Equal1/1 -> AND/1
  [VTQD_APSStaSys_enum] -> Equal4/1
  [VTQD_VehActSpd_kph] -> Relational Operator1/1
  AND1/1 -> NOT2/1, Timer/1  "VTQD_APSStasysLow_flg"
  Constant5/1 -> Equal4/2
  VTQD_VehActSpd_kph/1 -> [VTQD_VehActSpd_kph]
  VTQD_APSStaSys_enum/1 -> [VTQD_APSStaSys_enum]
  VTQD_AutiHoldRelease_flg/1 -> [VTQD_AutiHoldRelease_flg]
  task_time_s/1 -> [task_time_s]
  [VTQD_APSReqTimer_s] -> VTQD_APSReqTimer_s/1
  [VTQD_APSReq_enum] -> VTQD_APSReq_enum/1
  [VTQD_APSDecReqA_flg] -> VTQD_APSDecReqA_flg/1
  [VTQD_AutiHoldRelease_flg] -> NOT1/1
  VVMC_EstSlope_Deg/1 -> [VVMC_EstSlope_Deg]
  MTQD_APSReqLowSpd_Y_kph/1 -> Relational Operator1/2  "VTQD_APSReqLowSpd_kph"
  [VVMC_EstSlope_Deg] -> MTQD_APSReqLowSpd_Y_kph/1
  SR_Latch/1 -> AND1/1
  Relational Operator1/1 -> SR_Latch/1
  AND2/1 -> SR_Latch/2
  [VTQD_AutiHoldRelease_flg] -> AND2/1
  Constant3/1 -> Equal2/2
  [VTQD_APSStaSys_enum] -> Equal2/1
  Equal2/1 -> AND2/2
  [VVMC_EstSlope_Deg] -> Relay/1
  Relay/1 -> Switch/2  "VTQD_OPDHoldUpDown_flg"
  Constant1/1 -> Switch/1
  Constant10/1 -> Switch/3
  Switch/1 -> [VTQD_APSReqUpSpd_kph]  "VTQD_APSReqUpSpd_kph"
  Constant11/1 -> Equal6/2
  Equal6/1 -> [VTQD_OPDHoldLamp_flg]  "VTQD_OPDHoldLamp_flg"
  [VTQD_APSReqTimer_s] -> Equal6/1
  [VTQD_OPDHoldLamp_flg] -> VTQD_OPDHoldLamp_flg/1

== system tqd/TQD/TorqueDemand/TorqueModule/OPD Hold/Parking Requeest Backup ==
  VTQD_APSReq_enum : Inport
  VTQD_APSReqTimer_s : Inport  Port=2
  VTQD_ParkRequest_flg : Inport  Port=3
  task_time_s : Inport  Port=4
  VTQD_AutiHoldRelease_flg : Inport  Port=5
  AND : Logic  AllPortsSameDT=off  OutDataTypeStr=boolean
  AND1 : Logic  AllPortsSameDT=off  OutDataTypeStr=boolean
  AND3 : Logic  Inputs=3  AllPortsSameDT=off  OutDataTypeStr=boolean
  Constant1 : Constant  Value=KTQD_APSReqDelayTime_s
  Constant16 : Constant  OutDataTypeStr=uint8
  Constant17 : Constant  Value=TRUE  OutDataTypeStr=uint8
  Constant2 : Constant  Value=KTQD_APSReqDelayTime_s
  Constant3 : Constant  Value=KTQD_OPDHoldBrkSW_flg
  Constant4 : Constant  Value=KTQD_OPDHoldAllowPark_flg
  Constant5 : Constant  Value=KTQD_OPDHoldAllowPark_s
  Constant6 : Constant  Value=KTQD_OPDHoldAllowGearPSW_flg
  DelayEnable : hcu_lib/Basic_Blocks/DelayEnable
  Equal6 : RelationalOperator  Operator===  OutDataTypeStr=boolean  RndMeth=Simplest
  NOT : Logic  Operator=NOT  AllPortsSameDT=off  OutDataTypeStr=boolean
  OR : Logic  Operator=OR  AllPortsSameDT=off  OutDataTypeStr=boolean
  Relational Operator1 : RelationalOperator  OutDataTypeStr=boolean  RndMeth=Simplest
  Relational Operator6 : RelationalOperator  OutDataTypeStr=boolean  RndMeth=Simplest
  SR_Latch : hcu_lib/Basic_Blocks/SR_Latch
  Switch4 : Switch  Criteria=u2 > Threshold
  VTQD_ActParkRequest_flg : Outport
  VTQD_OPDHoldAllowPark_flg : Outport  Port=2
  wires:
  Constant3/1 -> AND3/2
  Constant1/1 -> Relational Operator6/2
  Equal6/1 -> AND3/1
  [VTQD_APSReq_enum] -> Equal6/1
  Relational Operator6/1 -> AND3/3
  [VTQD_ParkRequest_flg] -> Switch4/3
  Constant17/1 -> Switch4/1
  Constant16/1 -> Equal6/2
  Switch4/1 -> [VTQD_ActParkRequest_flg]  "VTQD_ActParkRequest_flg"
  [VTQD_APSReqTimer_s] -> Relational Operator6/1
  VTQD_APSReq_enum/1 -> [VTQD_APSReq_enum]
  VTQD_APSReqTimer_s/1 -> [VTQD_APSReqTimer_s]
  VTQD_ParkRequest_flg/1 -> [VTQD_ParkRequest_flg]
  [VTQD_ActParkRequest_flg] -> VTQD_ActParkRequest_flg/1
  Constant2/1 -> Relational Operator1/2
  [VTQD_APSReqTimer_s] -> Relational Operator1/1
  task_time_s/1 -> [task_time_s]
  AND/1 -> DelayEnable/1
  Relational Operator1/1 -> AND/1
  Constant4/1 -> AND/2
  Constant5/1 -> DelayEnable/2
  DelayEnable/1 -> SR_Latch/1
  [VTQD_AutiHoldRelease_flg] -> SR_Latch/2
  VTQD_AutiHoldRelease_flg/1 -> [VTQD_AutiHoldRelease_flg]
  SR_Latch/1 -> [VTQD_OPDHoldAllowPark_flg]  "VTQD_OPDHoldAllowPark_flg"
  OR/1 -> Switch4/2
  AND3/1 -> OR/1
  [task_time_s] -> DelayEnable/3
  [VTQD_OPDHoldAllowPark_flg] -> AND1/1
  AND1/1 -> OR/2
  NOT/1 -> AND1/2
  Constant6/1 -> NOT/1
  [VTQD_OPDHoldAllowPark_flg] -> VTQD_OPDHoldAllowPark_flg/1
